simulink model "correlator_complex_core"  (Simulink 7.1)
settings: Solver=ode45  StartTime=0.0  StopTime=10000  RelTol=1e-3
libraries: xbsIndex_r4 x252, cfa_library x72, casper_library_misc x7
(part 1 of 5)
settings Model: Creator=Administrator  LastModifiedBy=Rurik A Primiani

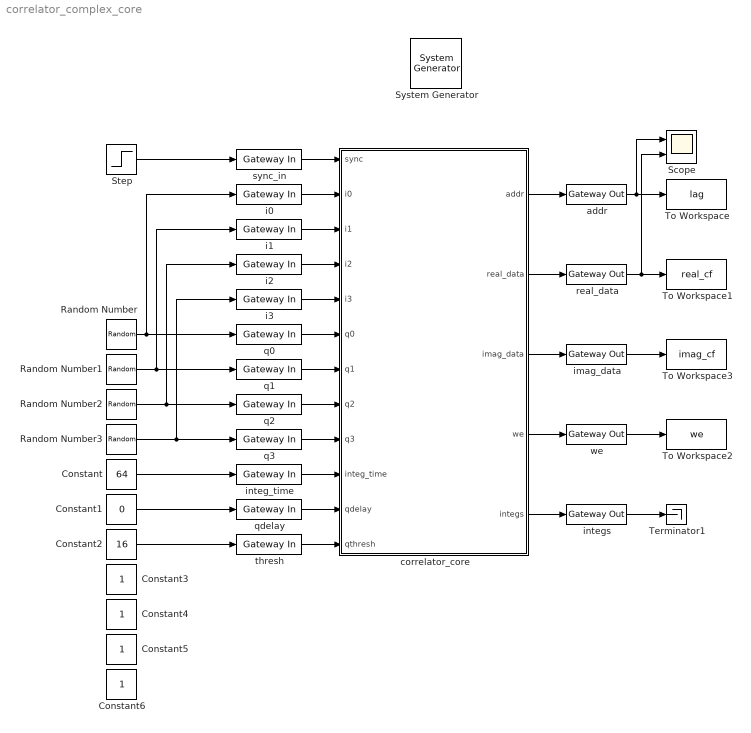
== system correlator_complex_core ==
  " System Generator" : xbsIndex_r4/ System Generator  Tag=genX  SystemSampleTime=-1  xilinxfamily=virtex2p  part=xc2vp50  speed=-7  package=ff1152  synthesis_tool=XST  clock_wrapper=Clock Enables  directory=./correlator_core  testbench=off  simulink_period=1  sysclk_period=100  dcm_input_clock_period=100  incr_netlist=off  trim_vbits=Everywhere in SubSystem  dbl_ovrd=According to Block Masks  core_generation=According to Block Masks  run_coregen=off  deprecated_control=off  eval_field=0  block_type=sysgen
      settings: block_version=10.1.3
  Constant : Constant  Value=64  OutDataType=sfix(16)  OutScaling=2^0
  Constant1 : Constant  Value=0  OutDataType=sfix(16)  OutScaling=2^0
  Constant2 : Constant  Value=16  OutDataType=sfix(16)  OutScaling=2^0
  Constant{3..6} (4 alike) : Constant  OutDataType=sfix(16)  OutScaling=2^0
  Random Number{,1..3} (4 alike) : RandomNumber  Variance=128  Seed=ceil(1000*rand())  SampleTime=0
  Scope : Scope  NumInputPorts=2
      settings: YMin=-5~-5  YMax=5~5
  Step : Step  Time=100  SampleTime=0
  Terminator1 : Terminator
  To Workspace : ToWorkspace  VariableName=lag  SampleTime=-1  SaveFormat=Array
  To Workspace1 : ToWorkspace  VariableName=real_cf  SampleTime=-1  SaveFormat=Array
  To Workspace2 : ToWorkspace  VariableName=we  SampleTime=-1  SaveFormat=Array
  To Workspace3 : ToWorkspace  VariableName=imag_cf  SampleTime=-1  SaveFormat=Array
  addr : xbsIndex_r4/Gateway Out  hdl_port=on  timing_constraint=None  locs_specified=off  LOCs={}  block_type=gatewayout
      settings: infoedit="Gateway out block.  Converts Xilinx fixed point inputs into ouputs of type Simulink integer, double, or fixed point.<P><P>Hardware notes:  In hardware these blocks become top level output ports or are discarded, depending on how they are configured."  block_version=10.1.3
  correlator_core : Subsystem
  i{0..3} (4 alike) : xbsIndex_r4/Gateway In  arith_type="Signed  (2's comp)"  n_bits=8  bin_pt=0  quantization=Truncate  overflow=Wrap  period=1  dbl_ovrd=off  timing_constraint=None  locs_specified=off  LOCs={}  block_type=gatewayin
      settings: infoedit="Gateway in block.  Converts inputs of type Simulink integer, double and fixed point to  Xilinx fixed point type.<br><br>Hardware notes:  In hardware these blocks become top level input ports."  block_version=10.1.3
  imag_data : xbsIndex_r4/Gateway Out  hdl_port=on  timing_constraint=None  locs_specified=off  LOCs={}  block_type=gatewayout
      settings: infoedit="Gateway out block.  Converts Xilinx fixed point inputs into ouputs of type Simulink integer, double, or fixed point.<P><P>Hardware notes:  In hardware these blocks become top level output ports or are discarded, depending on how they are configured."  block_version=10.1.3
  integ_time : xbsIndex_r4/Gateway In  arith_type=Unsigned  n_bits=32  bin_pt=0  quantization=Truncate  overflow=Wrap  period=1  dbl_ovrd=off  timing_constraint=None  locs_specified=off  LOCs={}  block_type=gatewayin
      settings: infoedit="Gateway in block.  Converts inputs of type Simulink integer, double and fixed point to  Xilinx fixed point type.<P><P>Hardware notes:  In hardware these blocks become top level input ports."  block_version=10.1.3
  integs : xbsIndex_r4/Gateway Out  hdl_port=on  timing_constraint=None  locs_specified=off  LOCs={}  block_type=gatewayout
      settings: infoedit="Gateway out block.  Converts Xilinx fixed point inputs into ouputs of type Simulink integer, double, or fixed point.<P><P>Hardware notes:  In hardware these blocks become top level output ports or are discarded, depending on how they are configured."  block_version=10.1.3
  q{0..3} (4 alike) : xbsIndex_r4/Gateway In  arith_type="Signed  (2's comp)"  n_bits=8  bin_pt=0  quantization=Truncate  overflow=Wrap  period=1  dbl_ovrd=off  timing_constraint=None  locs_specified=off  LOCs={}  block_type=gatewayin
      settings: infoedit="Gateway in block.  Converts inputs of type Simulink integer, double and fixed point to  Xilinx fixed point type.<br><br>Hardware notes:  In hardware these blocks become top level input ports."  block_version=10.1.3
  qdelay : xbsIndex_r4/Gateway In  arith_type=Unsigned  n_bits=11  bin_pt=0  quantization=Truncate  overflow=Wrap  period=1  dbl_ovrd=off  timing_constraint=None  locs_specified=off  LOCs={}  block_type=gatewayin
      settings: infoedit="Gateway in block.  Converts inputs of type Simulink integer, double and fixed point to  Xilinx fixed point type.<P><P>Hardware notes:  In hardware these blocks become top level input ports."  block_version=10.1.3
  real_data : xbsIndex_r4/Gateway Out  hdl_port=on  timing_constraint=None  locs_specified=off  LOCs={}  block_type=gatewayout
      settings: infoedit="Gateway out block.  Converts Xilinx fixed point inputs into ouputs of type Simulink integer, double, or fixed point.<P><P>Hardware notes:  In hardware these blocks become top level output ports or are discarded, depending on how they are configured."  block_version=10.1.3
  sync_in : xbsIndex_r4/Gateway In  arith_type=Boolean  n_bits=16  bin_pt=14  quantization="Round  (unbiased: +/- Inf)"  overflow=Saturate  period=1  dbl_ovrd=off  timing_constraint=None  locs_specified=off  LOCs={}  block_type=gatewayin
      settings: infoedit="Gateway in block.  Converts inputs of type Simulink integer, double and fixed point to  Xilinx fixed point type.<P><P>Hardware notes:  In hardware these blocks become top level input ports."  block_version=10.1.3
  thresh : xbsIndex_r4/Gateway In  arith_type=Unsigned  n_bits=7  bin_pt=0  quantization=Truncate  overflow=Wrap  period=1  dbl_ovrd=off  timing_constraint=None  locs_specified=off  LOCs={}  block_type=gatewayin
      settings: infoedit="Gateway in block.  Converts inputs of type Simulink integer, double and fixed point to  Xilinx fixed point type.<P><P>Hardware notes:  In hardware these blocks become top level input ports."  block_version=10.1.3
  we : xbsIndex_r4/Gateway Out  hdl_port=on  timing_constraint=None  locs_specified=off  LOCs={}  block_type=gatewayout
      settings: infoedit="Gateway out block.  Converts Xilinx fixed point inputs into ouputs of type Simulink integer, double, or fixed point.<P><P>Hardware notes:  In hardware these blocks become top level output ports or are discarded, depending on how they are configured."  block_version=10.1.3
  wires:
  sync_in/1 -> correlator_core/1(sync)
  i0/1 -> correlator_core/2(i0)
  i1/1 -> correlator_core/3(i1)
  i2/1 -> correlator_core/4(i2)
  i3/1 -> correlator_core/5(i3)
  q0/1 -> correlator_core/6(q0)
  q1/1 -> correlator_core/7(q1)
  q2/1 -> correlator_core/8(q2)
  q3/1 -> correlator_core/9(q3)
  Step/1 -> sync_in/1
  integ_time/1 -> correlator_core/10(integ_time)
  Constant/1 -> integ_time/1
  addr/1 -> To Workspace/1, Scope/1
  real_data/1 -> To Workspace1/1, Scope/2
  we/1 -> To Workspace2/1
  Constant1/1 -> qdelay/1
  qdelay/1 -> correlator_core/11(qdelay)
  thresh/1 -> correlator_core/12(qthresh)
  Constant2/1 -> thresh/1
  Random Number/1 -> q0/1, i0/1
  Random Number1/1 -> q1/1, i1/1
  Random Number2/1 -> q2/1, i2/1
  Random Number3/1 -> q3/1, i3/1
  correlator_core/1(addr) -> addr/1
  correlator_core/2(real_data) -> real_data/1
  imag_data/1 -> To Workspace3/1
  correlator_core/3(imag_data) -> imag_data/1
  correlator_core/4(we) -> we/1
  correlator_core/5(integs) -> integs/1
  integs/1 -> Terminator1/1

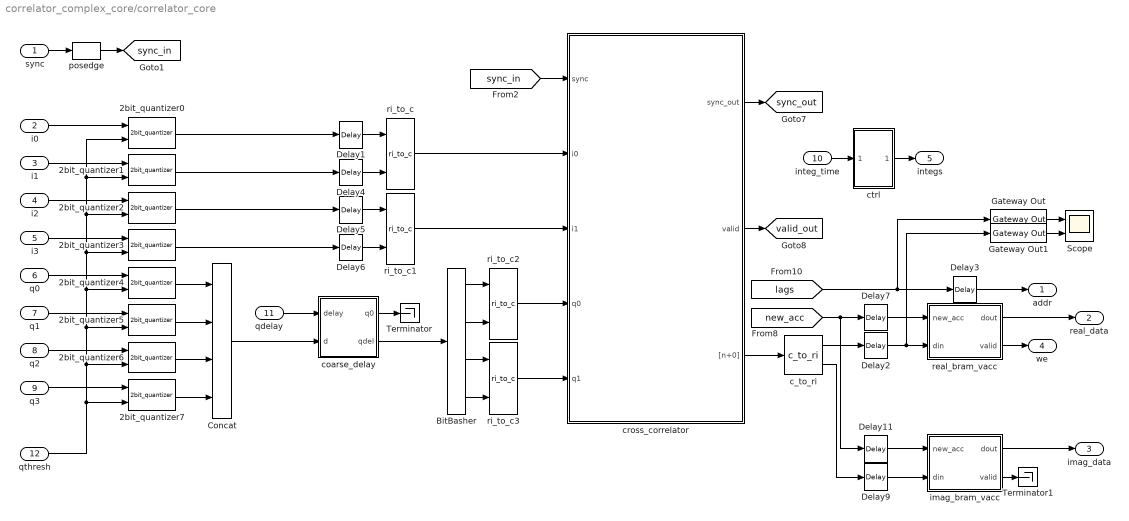
== system correlator_complex_core/correlator_core ==
  sync : Inport
  i0 : Inport  Port=2
  i1 : Inport  Port=3
  i2 : Inport  Port=4
  i3 : Inport  Port=5
  q0 : Inport  Port=6
  q1 : Inport  Port=7
  q2 : Inport  Port=8
  q3 : Inport  Port=9
  integ_time : Inport  Port=10
  qdelay : Inport  Port=11
  qthresh : Inport  Port=12
  2bit_quantizer{0..7} (8 alike) : cfa_library/2bit_quantizer  SystemSampleTime=-1  relational_delay=2  mux_delay=1
  BitBasher : xbsIndex_r4/BitBasher  bitexpr=|  display_expr=off  sr_1=1  arith_type1=Unsigned  bin_pt1=0  sr_2=2  arith_type2=Unsigned  bin_pt2=0  sr_3=3  arith_type3=Unsigned  bin_pt3=0  sr_4=4  arith_type4=Unsigned  bin_pt4=0  dbl_ovrd=off  block_type=bitbasher
      | <html><head><meta name="qrichtext" content="1" /><style type="text/css">
      | p, li { white-space: pre-wrap; }
      | </style></head><body style=" font-family:'MS Shell Dlg 2'; font-size:8.25pt; font-weight:400; font-style:normal;">
      | <p style=" margin-top:0px; margin-bottom:0px; margin-left:0px; margin-right:0px; -qt-block-indent:0; text-indent:0px; font-size:8pt;"><span style=" font-family:'MS Shell Dlg';">q0={i[7:6]}<br />q1={i[5:4]}<br />q2={i[3:2]}<br />q3={i[1:0]}<br /></span></p></body></html>
      settings: block_version=10.1.3
  Concat : xbsIndex_r4/Concat  num_inputs=4  dbl_ovrd=off  block_type=concat
      settings: block_version=10.1.3
  Delay{1,4..6} (4 alike) : xbsIndex_r4/Delay  en=off  latency=3  dbl_ovrd=off  reg_retiming=off  block_type=delay
      settings: block_version=11.4
  Delay{2,7,9,11} (4 alike) : xbsIndex_r4/Delay  en=off  latency=1  dbl_ovrd=off  reg_retiming=off  block_type=delay
      settings: block_version=11.4
  Delay3 : xbsIndex_r4/Delay  en=off  latency=0  dbl_ovrd=off  reg_retiming=off  block_type=delay
      settings: block_version=11.4
  Gateway Out : xbsIndex_r4/Gateway Out  hdl_port=on  timing_constraint=None  locs_specified=off  LOCs={}  block_type=gatewayout
      settings: infoedit="Gateway out block.  Converts Xilinx fixed point inputs into ouputs of type Simulink integer, double, or fixed point.<P><P>Hardware notes:  In hardware these blocks become top level output ports or are discarded, depending on how they are configured."  block_version=10.1.3
  Gateway Out1 : xbsIndex_r4/Gateway Out  hdl_port=on  timing_constraint=None  locs_specified=off  LOCs={}  block_type=gatewayout
      settings: infoedit="Gateway out block.  Converts Xilinx fixed point inputs into ouputs of type Simulink integer, double, or fixed point.<P><P>Hardware notes:  In hardware these blocks become top level output ports or are discarded, depending on how they are configured."  block_version=10.1.3
  Scope : Scope  NumInputPorts=2
      settings: YMin=-5~-5  YMax=5~5
  Terminator : Terminator
  Terminator1 : Terminator
  c_to_ri : casper_library_misc/c_to_ri  SystemSampleTime=-1  n_bits=11  bin_pt=0
      settings: AttributesFormatString=11_0 r/i
  coarse_delay : Subsystem
  cross_correlator : Subsystem  AncestorBlock=cfa_library/cross_correlator  mask(cross_correlator){total_lags=4, n_inputs=1, use_2bit=on, complex_in=on, input_bit_width=8, input_bin_pt=7, specify_data_type=off, output_bit_width=16, output_bin_pt=14, quantization=Truncate, overflow=Wrap, specify_mult=off, mult_spec=Behavioral, specify_add=off, add_spec=Fabric, mult_delay=3, add_delay=2, overall_delay=2, single_output=on}
      mask prompts: total_lags "Total Lags Centered at Zero: (2^?)"; n_inputs "Number of Simultaneous Inputs: (2^?)"; use_2bit "Use special 2-bit binary encoding"; complex_in "Complex inputs"; input_bit_width "Input Bit Width:"; input_bin_pt "Input Binary Point:"; specify_data_type "Specify output data type"; output_bit_width "Output Bit Width:"; output_bin_pt "Output Binary Point:"; quantization "Quantization Behavior:"; overflow "Overflow Behavior"; specify_mult "Specify multiplier use (behavioural HDL if not specified)"; mult_spec "Multiplier specification:"; specify_add "Specify adder use (behavioural HDL if not specified)"; add_spec "Adder specification:"; mult_delay "Mult Latency:"; add_delay "Add Latency:"; overall_delay "Overall latency:"; single_output "Provide single output stream"
      mask help: This time-domain cross correlator accepts two real time-series and outputs the cross-correlation function for the given set of lags. The output is accumulated so that for every two input samples there is exactly one output sample.
      mask init:
      | cross_correlator_init(gcb,...
      |     'total_lags', total_lags,...
      |     'n_inputs', n_inputs,...
      |     'use_2bit', use_2bit,...
      |     'input_bit_width', input_bit_width,...
      |     'input_bin_pt', input_bin_pt,...
      |     'complex_in', complex_in,...
      |     'specify_data_type', specify_data_type,...
      |     'output_bit_width', output_bit_width,...
      |     'output_bin_pt', output_bin_pt,...
      |     'quantization', quantization,...
      |     'overflow', overflow,...
      |     'specify_mult', specify_mult,...
      |     'mult_spec', mult_spec,...
      |     'specify_add', specify_add,...
      |     'add_spec', add_spec,...
      |     'mult_delay', mult_delay,...
      |     'add_delay', add_delay,...
      |     'overall_delay', overall_delay,...
      |     'single_output', single_output);
      settings: AttributesFormatString=|
      | 16 lags, Demux: 2, Outputs: 1
      | Special 2-bit complex binary encoding
      |  Mult: Behavioral, Add: Fabric
      mask StyleString: edit,edit,checkbox,checkbox,edit,edit,checkbox,edit,edit,popup(Truncate|Round (unbiased: +/- Inf)|Round (unbiased: Even Values)),popup(Wrap|Saturate|Flag as error),checkbox,popup(Behavioral|Core|Embedded),checkbox,popup(Fabric|DSP48),edit,edit,edit,checkbox
      mask CallbackString:
      | ||use_2bit = get_param(gcb,'use_2bit');
      | enables = get_param(gcb, 'MaskEnables');
      | if( strcmp(use_2bit,'on')),
      |     enables{4} = 'on';
      |     enables{5} = 'off';
      |     enables{6} = 'off';
      | else
      |     enables{4} = 'off';
      |     enables{5} = 'on';
      |     enables{6} = 'on';
      | end
      | set_param(gcb, 'MaskEnables', enables);
      | ||||specify_data_type = get_param(gcb,'specify_data_type');
      | enables = get_param(gcb, 'MaskEnables');
      | if( strcmp(specify_data_type,'off')),
      |     enables{8} = 'off';
      |     enables{9} = 'off';
      |     enables{10} = 'off';
      |     enables{11} = 'off';
      | else
      |     enables{8} = 'on';
      |     enables{9} = 'on';
      |     enables{10} = 'on';
      |     enables{11} = 'on';
      | end
      | set_param(gcb, 'MaskEnables', enables);
      | |||||specify_mult = get_param(gcb,'specify_mult');
      | enables = get_param(gcb, 'MaskEnables');
      | if( strcmp(specify_mult,'off')),
      |     enables{13} = 'off';
      | else
      |     enables{13} = 'on';
      | end
      | set_param(gcb, 'MaskEnables', enables);
      | ||specify_add = get_param(gcb,'specify_add');
      | enables = get_param(gcb, 'MaskEnables');
      | if( strcmp(specify_add,'off')),
      |     enables{15} = 'off';
      | else
      |     enables{15} = 'on';
      | end
      | set_param(gcb, 'MaskEnables', enables);
      | |||||
      mask TabNameString: Basic,Basic,Input,Input,Input,Input,Output,Output,Output,Output,Output,Implementation,Implementation,Implementation,Implementation,Implementation,Implementation,Implementation,Basic
  ctrl : Subsystem  mask{total_lags=4}
      mask prompts: total_lags "Total Lags (2^?):"
      mask Display: fprintf('CTRL');
  imag_bram_vacc : Subsystem  mask(simple_bram_vacc){vec_len=16, arith_type=Signed, n_bits=32, bin_pt=0, add_latency=3}
      mask prompts: vec_len "Vector length:"; arith_type "Output type:"; n_bits "Bit width (output):"; bin_pt "Binary point (output):"; add_latency "Adder latency:"
      mask help: This simple vector accumulator is based on a shift register. It outputs its previous accumulated vector after a new_acc pulse is received.
      mask init:
      | simple_bram_vacc_init(gcb, ...
      |     'vec_len', vec_len, ...
      |     'arith_type', arith_type, ...
      |     'n_bits', n_bits, ...
      |     'bin_pt', bin_pt);
      mask StyleString: edit,popup(Signed|Unsigned),edit,edit,edit
  posedge : casper_library_misc/posedge  Tag=Rising Edge Detector  SystemSampleTime=-1
  real_bram_vacc : Subsystem  mask(simple_bram_vacc){vec_len=16, arith_type=Signed, n_bits=32, bin_pt=0, add_latency=3}
      mask prompts: vec_len "Vector length:"; arith_type "Output type:"; n_bits "Bit width (output):"; bin_pt "Binary point (output):"; add_latency "Adder latency:"
      mask help: This simple vector accumulator is based on a shift register. It outputs its previous accumulated vector after a new_acc pulse is received.
      mask init:
      | simple_bram_vacc_init(gcb, ...
      |     'vec_len', vec_len, ...
      |     'arith_type', arith_type, ...
      |     'n_bits', n_bits, ...
      |     'bin_pt', bin_pt);
      mask StyleString: edit,popup(Signed|Unsigned),edit,edit,edit
  ri_to_c{,1..3} (4 alike) : casper_library_misc/ri_to_c  SystemSampleTime=-1
  addr : Outport
  real_data : Outport  Port=2
  imag_data : Outport  Port=3
  we : Outport  Port=4
  integs : Outport  Port=5
  tag scope: sync_in=global, sync_out=global, valid_out=global
  wires:
  Delay2/1 -> real_bram_vacc/2(din), Gateway Out1/1
  [lags] -> Delay3/1, Gateway Out/1
  [new_acc] -> Delay7/1, Delay11/1
  real_bram_vacc/1(dout) -> real_data/1
  sync/1 -> posedge/1
  Delay3/1 -> addr/1
  real_bram_vacc/2(valid) -> we/1
  integ_time/1 -> ctrl/1(integ_time)
  ctrl/1(integs) -> integs/1
  posedge/1 -> [sync_in]
  2bit_quantizer4/1 -> Concat/1
  2bit_quantizer5/1 -> Concat/2
  2bit_quantizer6/1 -> Concat/3
  2bit_quantizer7/1 -> Concat/4
  2bit_quantizer0/1 -> Delay1/1
  2bit_quantizer1/1 -> Delay4/1
  2bit_quantizer2/1 -> Delay5/1
  2bit_quantizer3/1 -> Delay6/1
  i0/1 -> 2bit_quantizer0/1
  i1/1 -> 2bit_quantizer1/1
  i2/1 -> 2bit_quantizer2/1
  i3/1 -> 2bit_quantizer3/1
  q0/1 -> 2bit_quantizer4/1
  q1/1 -> 2bit_quantizer5/1
  q2/1 -> 2bit_quantizer6/1
  q3/1 -> 2bit_quantizer7/1
  cross_correlator/1(sync_out) -> [sync_out]
  cross_correlator/2(valid) -> [valid_out]
  [sync_in] -> cross_correlator/1(sync)
  coarse_delay/2(qdel) -> BitBasher/1
  qdelay/1 -> coarse_delay/1(delay)
  Concat/1 -> coarse_delay/2(d)
  qthresh/1 -> 2bit_quantizer0/2, 2bit_quantizer1/2, 2bit_quantizer2/2, 2bit_quantizer3/2, 2bit_quantizer4/2, 2bit_quantizer5/2, 2bit_quantizer6/2, 2bit_quantizer7/2
  coarse_delay/1(q0) -> Terminator/1
  Delay7/1 -> real_bram_vacc/1(new_acc)
  Delay1/1 -> ri_to_c/1
  Delay4/1 -> ri_to_c/2
  ri_to_c/1 -> cross_correlator/2(i0)
  Delay5/1 -> ri_to_c1/1
  Delay6/1 -> ri_to_c1/2
  ri_to_c1/1 -> cross_correlator/3(i1)
  ri_to_c2/1 -> cross_correlator/4(q0)
  BitBasher/1 -> ri_to_c2/1
  BitBasher/2 -> ri_to_c2/2
  BitBasher/3 -> ri_to_c3/1
  BitBasher/4 -> ri_to_c3/2
  ri_to_c3/1 -> cross_correlator/5(q1)
  c_to_ri/1 -> Delay2/1
  cross_correlator/3("[n+0]") -> c_to_ri/1
  Delay9/1 -> imag_bram_vacc/2(din)
  imag_bram_vacc/1(dout) -> imag_data/1
  Delay11/1 -> imag_bram_vacc/1(new_acc)
  c_to_ri/2 -> Delay9/1
  imag_bram_vacc/2(valid) -> Terminator1/1
  Gateway Out/1 -> Scope/1
  Gateway Out1/1 -> Scope/2

== system correlator_complex_core/correlator_core/coarse_delay ==
  delay : Inport
  d : Inport  Port=2
  AddSub2 : xbsIndex_r4/AddSub  mode=Subtraction  use_carryin=off  use_carryout=off  en=off  latency=2  precision=User Defined  arith_type=Unsigned  n_bits=11  bin_pt=0  quantization=Truncate  overflow=Wrap  dbl_ovrd=off  use_behavioral_HDL=off  pipelined=on  use_rpm=on  hw_selection=Fabric  block_type=addsub
      settings: block_version=10.1.3
  Constant : xbsIndex_r4/Constant  arith_type=Boolean  const=1  n_bits=16  bin_pt=14  explicit_period=on  period=1  equ=P=C  opselect=C  inp2=PCIN>>17  opr=+  inp1=P  carry=CIN  dbl_ovrd=off  block_type=constant
  Constant1 : xbsIndex_r4/Constant  arith_type=Boolean  const=0  n_bits=16  bin_pt=14  explicit_period=on  period=1  equ=P=C  opselect=C  inp2=PCIN>>17  opr=+  inp1=P  carry=CIN  dbl_ovrd=off  block_type=constant
  Constant3 : xbsIndex_r4/Constant  arith_type=Unsigned  const=0  n_bits=8  bin_pt=0  explicit_period=on  period=1  equ=P=C  opselect=C  inp2=PCIN>>17  opr=+  inp1=P  carry=CIN  dbl_ovrd=off  block_type=constant
  Counter : xbsIndex_r4/Counter  cnt_type=Free Running  cnt_to=Inf  operation=Up  start_count=0  cnt_by_val=1  arith_type=Unsigned  n_bits=11  bin_pt=0  load_pin=off  rst=off  en=off  explicit_period=on  period=1  dbl_ovrd=off  use_behavioral_HDL=off  use_rpm=off  implementation=Fabric  block_type=counter
  dpr16 : xbsIndex_r4/Dual Port RAM  depth=2048  initVector=zeros(1,2048)  distributed_mem=Block RAM  init_a=0  init_b=0  rst_a=off  rst_b=off  en_a=off  en_b=off  latency=1  write_mode_A=No Read On Write  write_mode_B=Read After Write  dbl_ovrd=off  optimize=Speed  use_rpm=on  block_type=dpram
      settings: block_version=10.1.3
  q0 : Outport
  qdel : Outport  Port=2
  wires:
  Counter/1 -> AddSub2/1, dpr16/1
  AddSub2/1 -> dpr16/4
  Constant/1 -> dpr16/3
  Constant1/1 -> dpr16/6
  Constant3/1 -> dpr16/5
  d/1 -> dpr16/2
  dpr16/1 -> q0/1
  delay/1 -> AddSub2/2
  dpr16/2 -> qdel/1
